simulink model "pFIR_Testing"  (R2019b)
settings: Solver=FixedStepDiscrete  StartTime=0.0  StopTime=stop_time  RelTol=1e-3
InitFcn:
  | pwd
  | sm_callback_init
StopFcn:
  | sm_callback_stop
values from neighbouring files (symbols this model uses):
  mp = sm_stop_process_output(mp)    [sm_callback_stop.m]
libraries: simulink x3, FPGA_Open_Speech_Tools x2
settings Model: Creator=Ross  LastModifiedBy=Balad
settings DataIOCC: ReturnWorkspaceOutputs=off
settings OptimizationCC: BlockReduction=off  ConditionallyExecuteInputs=off  DefaultParameterBehavior=Inlined
settings DebuggingCC: ReadBeforeWriteMsg=DisableAll  WriteAfterWriteMsg=DisableAll  WriteAfterReadMsg=DisableAll  AlgebraicLoopMsg=error  MultiTaskDSMMsg=none  SingleTaskRateTransMsg=error  PregeneratedLibrarySubsystemCodeDiagnostic=none  ArithmeticOperatorsInVariantConditions=warning
settings HardwareCC: ProdBitPerPointer=32  ProdBitPerSizeT=32  ProdBitPerPtrDiffT=32  ProdLargestAtomicFloat=None  ProdIntDivRoundTo=Undefined  ProdEndianess=Unspecified  ProdWordSize=32  ProdHWDeviceType=ASIC/FPGA->ASIC/FPGA  TargetBitPerPointer=64  TargetBitPerSizeT=64  TargetBitPerPtrDiffT=64  TargetLongLongMode=on  TargetIntDivRoundTo=Zero  TargetEndianess=LittleEndian  TargetWordSize=64  TargetHWDeviceType=Custom Processor->MATLAB Host Computer  ProdEqTarget=off
settings ModelReferenceCC: UpdateModelReferenceTargets=IfOutOfDate
settings SFSimCC: SFSimEcho=off  SimUseLocalCustomCode=off  CustomCodeUndefinedFunction=UseInterfaceOnly
settings RTWCC: RTWUseLocalCustomCode=off

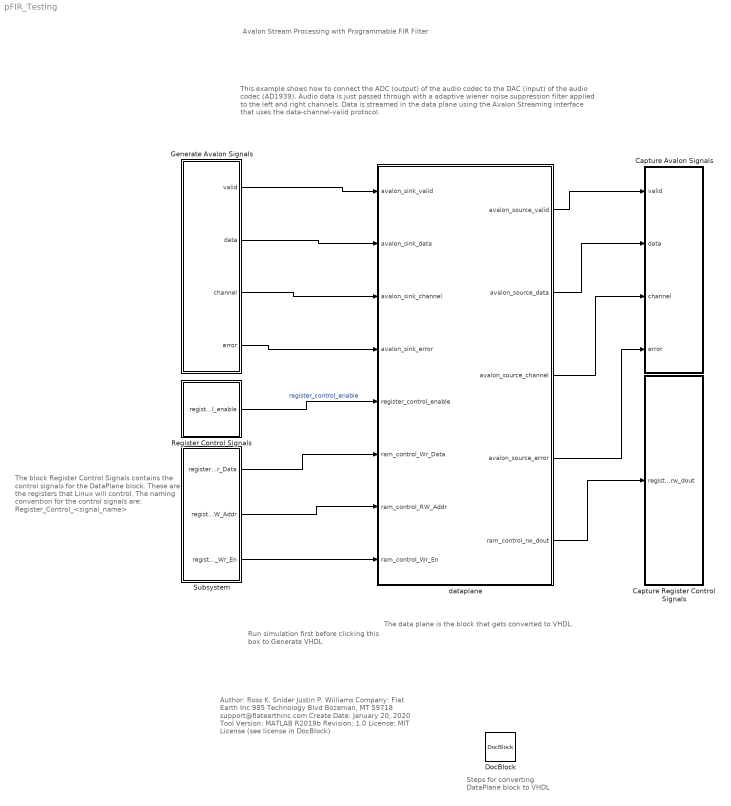
== system pFIR_Testing ==
  note: The data plane is the block that gets converted to VHDL.
  note: Author:          Ross K. Snider
      |                      Justin P. Williams
      | Company:     Flat Earth Inc
      |                       985 Technology Blvd
      |                       Bozeman, MT 59718
      |                       support@flatearthinc.com
      | Create Date:  January 20, 2020
      | Tool Version:  MATLAB R2019b
      | Revision:        1.0
      | License:          MIT License (see license in DocBlock)
  note: This example shows how to connect the ADC (output) of the audio codec to the DAC (input) of the audio codec (AD1939). Audio data is just passed through with a adaptive wiener noise suppression filter applied to the left and right channels. Data is streamed in the data plane using the Avalon Streaming interface that uses the data-channel-valid protocol.
  note: Steps for converting
      | DataPlane block
      | to VHDL
  note: Avalon Stream Processing
      | with Programmable FIR Filter
  note: Run simulation first
      | before clicking this box to
      | Generate VHDL
  note: The block Register Control Signals contains
      | the control signals for the DataPlane block.
      | These are the registers that Linux will control.
      | The naming convention for the control
      | signals are:  Register_Control_<signal_name>
  Capture Avalon Signals : Subsystem
  Capture Register Control Signals : Subsystem
  DocBlock : simulink/Model-Wide Utilities/DocBlock  DocumentType=HTML
  Generate Avalon Signals : Subsystem
  Register Control Signals : Subsystem
  Subsystem : Subsystem
  dataplane : Subsystem  TreatAsAtomicUnit=on
  wires:
  Generate Avalon Signals/2(data) -> dataplane/2(avalon_sink_data)
  Generate Avalon Signals/1(valid) -> dataplane/1(avalon_sink_valid)
  Generate Avalon Signals/3(channel) -> dataplane/3(avalon_sink_channel)
  Generate Avalon Signals/4(error) -> dataplane/4(avalon_sink_error)
  dataplane/2(avalon_source_data) -> Capture Avalon Signals/2(data)
  dataplane/1(avalon_source_valid) -> Capture Avalon Signals/1(valid)
  dataplane/3(avalon_source_channel) -> Capture Avalon Signals/3(channel)
  dataplane/4(avalon_source_error) -> Capture Avalon Signals/4(error)
  Register Control Signals/1(register_control_enable) -> dataplane/5(register_control_enable)  "register_control_enable"
  Subsystem/1(register_control_Wr_Data) -> dataplane/6(ram_control_Wr_Data)
  Subsystem/2(register_control_RW_Addr) -> dataplane/7(ram_control_RW_Addr)
  Subsystem/3(register_control_Wr_En) -> dataplane/8(ram_control_Wr_En)
  dataplane/5(ram_control_rw_dout) -> Capture Register Control Signals/1(register_control_rw_dout)

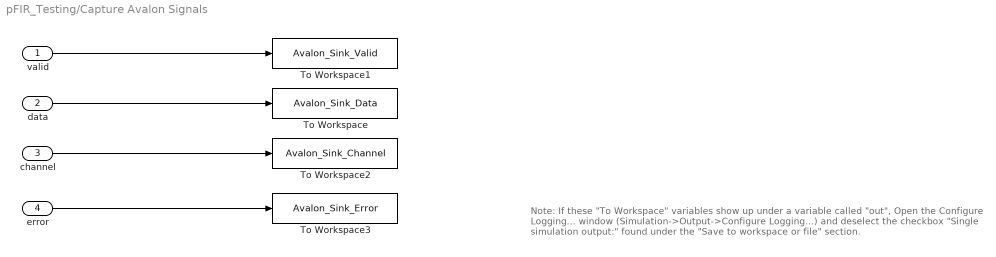
== system pFIR_Testing/Capture Avalon Signals ==
  note: Note:  If these "To Workspace" variables show up under a variable called "out",
      | Open the Configure Logging... window (Simulation->Output->Configure Logging...)
      | and deselect the checkbox "Single simulation output:" found under the "Save to workspace or file" section.
  valid : Inport
  data : Inport  Port=2
  channel : Inport  Port=3
  error : Inport  Port=4
  To Workspace : ToWorkspace  VariableName=Avalon_Sink_Data  SaveFormat=Timeseries  SampleTime=-1
  To Workspace1 : ToWorkspace  VariableName=Avalon_Sink_Valid  SaveFormat=Timeseries  SampleTime=-1
  To Workspace2 : ToWorkspace  VariableName=Avalon_Sink_Channel  SaveFormat=Timeseries  SampleTime=-1
  To Workspace3 : ToWorkspace  VariableName=Avalon_Sink_Error  SaveFormat=Timeseries  SampleTime=-1
  wires:
  data/1 -> To Workspace/1
  valid/1 -> To Workspace1/1
  error/1 -> To Workspace3/1
  channel/1 -> To Workspace2/1

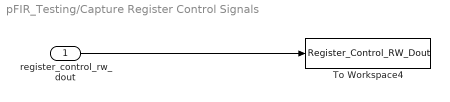
== system pFIR_Testing/Capture Register Control Signals ==
  register_control_rw_dout : Inport
  To Workspace4 : ToWorkspace  VariableName=Register_Control_RW_Dout  SaveFormat=Timeseries  SampleTime=-1
  wires:
  register_control_rw_dout/1 -> To Workspace4/1

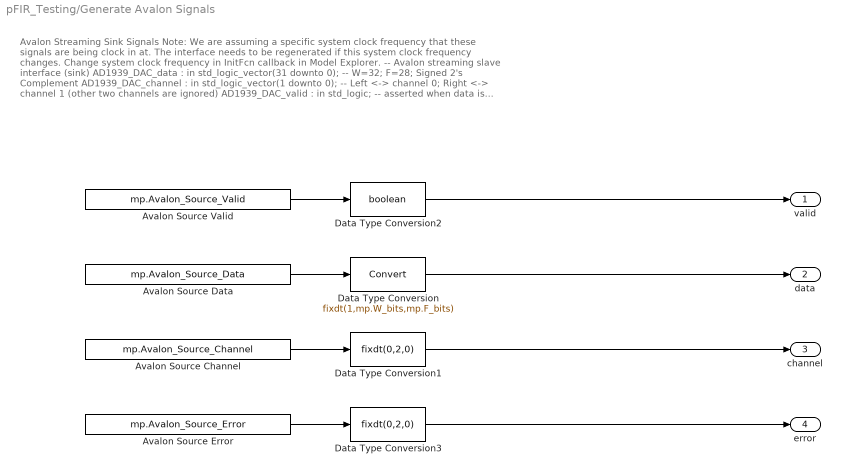
== system pFIR_Testing/Generate Avalon Signals ==
  note: Avalon Streaming Sink Signals
      | Note: We are assuming a specific system clock frequency that these signals are being clock in at.
      | The interface needs to be regenerated if this system clock frequency changes. Change system clock frequency in InitFcn callback in Model Explorer.
      |
      | -- Avalon streaming slave interface (sink)
      | AD1939_DAC_data : in std_logic_vector(31 downto 0); -- W=32; F=28; Signed 2's Complement
      | AD1939_DAC_channel : in std_logic_vector(1 downto 0); -- Left <-> channel 0; Right <-> channel 1 (other two channels are ignored)
      | AD1939_DAC_valid : in std_logic; -- asserted when data is valid
      | AD1939_DAC_error : in std_logic_vector(1 downto 0) -- error channel is ignored, assumed to be error free at this point
      |
      | For more information on the data-channel-valid protocol, s ee chapter 5 in Intel's Avalon Interfaced Specification (p. 40) at https://www.intel.com/content/dam/www/programmable/us/en/pdfs/literature/manual/mnl_avalon_spec.pdf
  Avalon Source Channel : FromWorkspace  VariableName=mp.Avalon_Source_Channel  OutDataTypeStr=double  SampleTime=mp.Ts_system
  "Avalon Source Data " : FromWorkspace  VariableName=mp.Avalon_Source_Data  OutDataTypeStr=double  SampleTime=mp.Ts_system
  Avalon Source Error : FromWorkspace  VariableName=mp.Avalon_Source_Error  OutDataTypeStr=double  SampleTime=mp.Ts_system
  Avalon Source Valid : FromWorkspace  VariableName=mp.Avalon_Source_Valid  OutDataTypeStr=double  SampleTime=mp.Ts_system
  Data Type Conversion : DataTypeConversion  OutDataTypeStr=fixdt(1,mp.W_bits,mp.F_bits)
  Data Type Conversion1 : DataTypeConversion  OutDataTypeStr=fixdt(0,2,0)
  Data Type Conversion2 : DataTypeConversion  OutDataTypeStr=boolean
  Data Type Conversion3 : DataTypeConversion  OutDataTypeStr=fixdt(0,2,0)
  valid : Outport  VectorParamsAs1DForOutWhenUnconnected=off
  data : Outport  Port=2  VectorParamsAs1DForOutWhenUnconnected=off
  channel : Outport  Port=3  VectorParamsAs1DForOutWhenUnconnected=off
  error : Outport  Port=4  VectorParamsAs1DForOutWhenUnconnected=off
  wires:
  Data Type Conversion1/1 -> channel/1
  Data Type Conversion2/1 -> valid/1
  Avalon Source Error/1 -> Data Type Conversion3/1
  Data Type Conversion/1 -> data/1
  Avalon Source Valid/1 -> Data Type Conversion2/1
  Data Type Conversion3/1 -> error/1
  Avalon Source Channel/1 -> Data Type Conversion1/1
  "Avalon Source Data "/1 -> Data Type Conversion/1

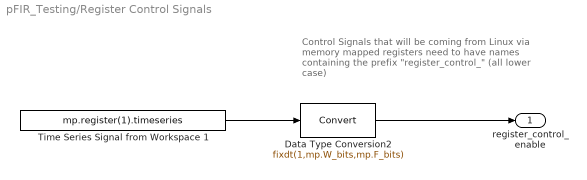
== system pFIR_Testing/Register Control Signals ==
  note: Control Signals that will be coming from Linux via
      | memory mapped registers need to have names
      | containing the prefix "register_control_"
      | (all lower case)
  Data Type Conversion2 : DataTypeConversion  OutDataTypeStr=fixdt(1,mp.W_bits,mp.F_bits)
  Time Series Signal from Workspace 1 : FromWorkspace  VariableName=mp.register(1).timeseries  OutDataTypeStr=double  SampleTime=mp.Ts_system  OutputAfterFinalValue=Holding final value
  register_control_enable : Outport  VectorParamsAs1DForOutWhenUnconnected=off
  wires:
  Time Series Signal from Workspace 1/1 -> Data Type Conversion2/1
  Data Type Conversion2/1 -> register_control_enable/1

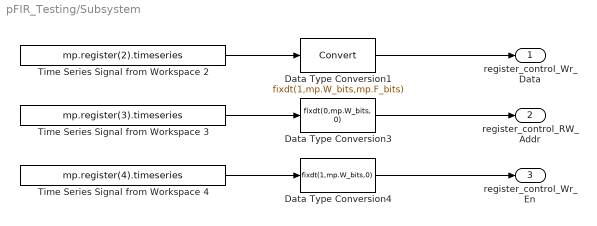
== system pFIR_Testing/Subsystem ==
  Data Type Conversion1 : DataTypeConversion  OutDataTypeStr=fixdt(1,mp.W_bits,mp.F_bits)
  Data Type Conversion3 : DataTypeConversion  OutDataTypeStr=fixdt(0,mp.W_bits, 0)
  Data Type Conversion4 : DataTypeConversion  OutDataTypeStr=fixdt(1,mp.W_bits,0)
  Time Series Signal from Workspace 2 : FromWorkspace  VariableName=mp.register(2).timeseries  OutDataTypeStr=double  SampleTime=mp.Ts_system
  Time Series Signal from Workspace 3 : FromWorkspace  VariableName=mp.register(3).timeseries  OutDataTypeStr=double  SampleTime=mp.Ts_system
  Time Series Signal from Workspace 4 : FromWorkspace  VariableName=mp.register(4).timeseries  OutDataTypeStr=double  SampleTime=mp.Ts_system
  register_control_Wr_Data : Outport  VectorParamsAs1DForOutWhenUnconnected=off
  register_control_RW_Addr : Outport  Port=2  VectorParamsAs1DForOutWhenUnconnected=off
  register_control_Wr_En : Outport  Port=3  VectorParamsAs1DForOutWhenUnconnected=off
  wires:
  Data Type Conversion1/1 -> register_control_Wr_Data/1
  Time Series Signal from Workspace 4/1 -> Data Type Conversion4/1
  Data Type Conversion3/1 -> register_control_RW_Addr/1
  Data Type Conversion4/1 -> register_control_Wr_En/1
  Time Series Signal from Workspace 3/1 -> Data Type Conversion3/1
  Time Series Signal from Workspace 2/1 -> Data Type Conversion1/1

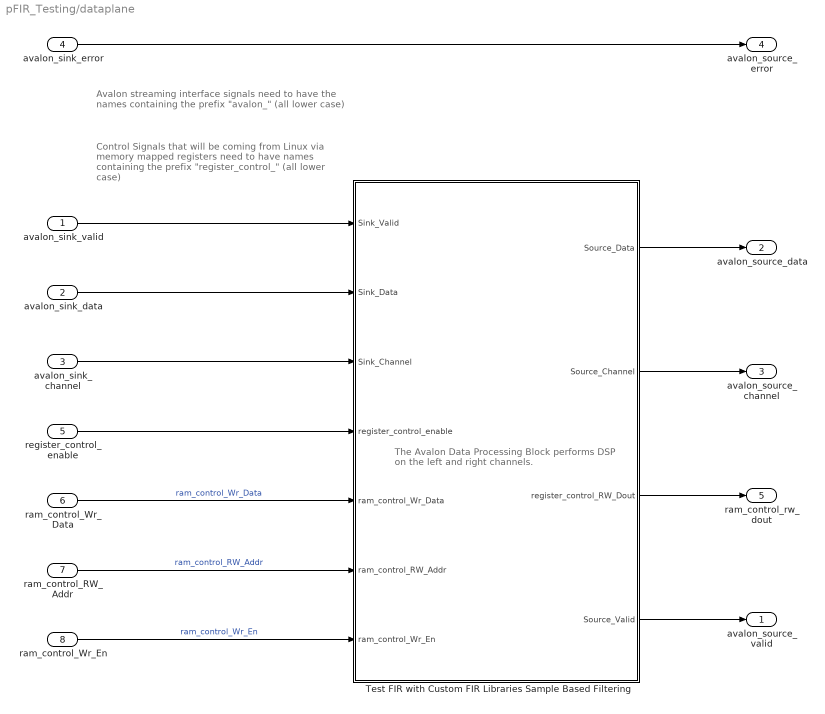
== system pFIR_Testing/dataplane ==
  note: Control Signals that will be coming from Linux via
      | memory mapped registers need to have names
      | containing the prefix "register_control_"
      | (all lower case)
  note: The Avalon Data Processing Block
      | performs DSP on the left and right channels.
  note: Avalon streaming interface signals need to have the
      | names containing the prefix "avalon_"
      | (all lower case)
  avalon_sink_valid : Inport
  avalon_sink_data : Inport  Port=2
  avalon_sink_channel : Inport  Port=3
  avalon_sink_error : Inport  Port=4
  register_control_enable : Inport  Port=5
  ram_control_Wr_Data : Inport  Port=6
  ram_control_RW_Addr : Inport  Port=7
  ram_control_Wr_En : Inport  Port=8
  Test FIR with Custom FIR Libraries Sample Based Filtering : Subsystem
  avalon_source_valid : Outport  VectorParamsAs1DForOutWhenUnconnected=off
  avalon_source_data : Outport  Port=2  VectorParamsAs1DForOutWhenUnconnected=off
  avalon_source_channel : Outport  Port=3  VectorParamsAs1DForOutWhenUnconnected=off
  avalon_source_error : Outport  Port=4  VectorParamsAs1DForOutWhenUnconnected=off
  ram_control_rw_dout : Outport  Port=5  VectorParamsAs1DForOutWhenUnconnected=off
  wires:
  avalon_sink_error/1 -> avalon_source_error/1
  Test FIR with Custom FIR Libraries Sample Based Filtering/1(Source_Data) -> avalon_source_data/1
  avalon_sink_valid/1 -> Test FIR with Custom FIR Libraries Sample Based Filtering/1(Sink_Valid)
  avalon_sink_data/1 -> Test FIR with Custom FIR Libraries Sample Based Filtering/2(Sink_Data)
  Test FIR with Custom FIR Libraries Sample Based Filtering/2(Source_Channel) -> avalon_source_channel/1
  avalon_sink_channel/1 -> Test FIR with Custom FIR Libraries Sample Based Filtering/3(Sink_Channel)
  register_control_enable/1 -> Test FIR with Custom FIR Libraries Sample Based Filtering/4(register_control_enable)
  ram_control_Wr_Data/1 -> Test FIR with Custom FIR Libraries Sample Based Filtering/5(ram_control_Wr_Data)  "ram_control_Wr_Data"
  ram_control_RW_Addr/1 -> Test FIR with Custom FIR Libraries Sample Based Filtering/6(ram_control_RW_Addr)  "ram_control_RW_Addr"
  ram_control_Wr_En/1 -> Test FIR with Custom FIR Libraries Sample Based Filtering/7(ram_control_Wr_En)  "ram_control_Wr_En"
  Test FIR with Custom FIR Libraries Sample Based Filtering/3(register_control_RW_Dout) -> ram_control_rw_dout/1
  Test FIR with Custom FIR Libraries Sample Based Filtering/4(Source_Valid) -> avalon_source_valid/1

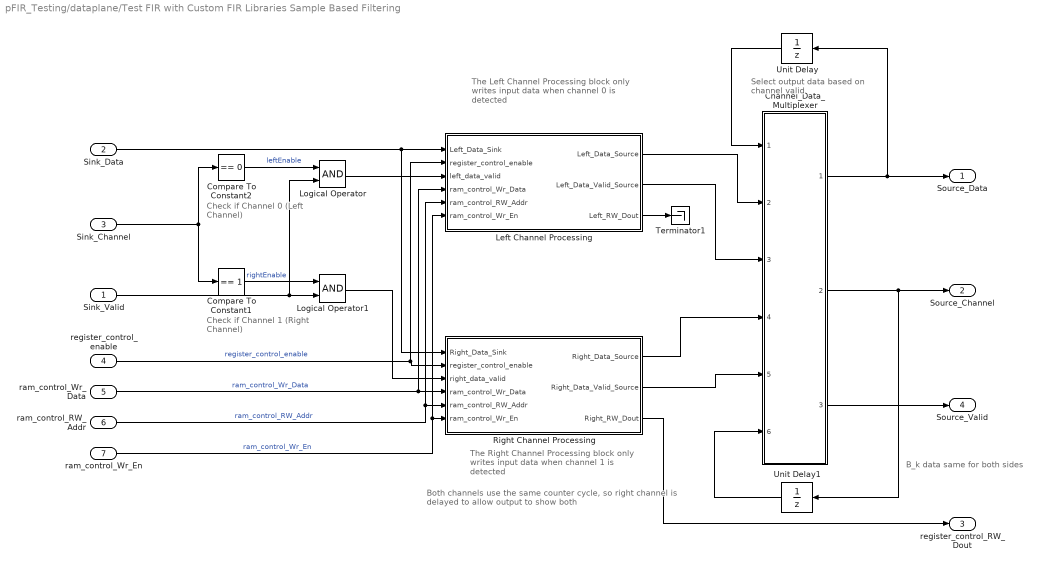
== system pFIR_Testing/dataplane/Test FIR with Custom FIR Libraries Sample Based Filtering ==
  note: B_k data same for both sides
  note: Both channels use the same counter cycle, so right channel
      | is delayed to allow output to show both
  note: The Left Channel Processing block
      | only writes input data when channel 0
      | is detected
  note: The Right Channel Processing block
      | only writes input data when channel 1
      | is detected
  note: Check if Channel 0
      | (Left Channel)
  note: Select output data
      | based on channel valid
  note: Check if Channel 1
      | (Right Channel)
  Sink_Valid : Inport
  Sink_Data : Inport  Port=2
  Sink_Channel : Inport  Port=3
  register_control_enable : Inport  Port=4
  ram_control_Wr_Data : Inport  Port=5
  ram_control_RW_Addr : Inport  Port=6
  ram_control_Wr_En : Inport  Port=7
  Channel_Data_Multiplexer : MATLAB Function  TreatAsAtomicUnit=on
  Compare To Constant1 : simulink/Logic and Bit Operations/Compare To Constant  relop===  const=1  OutDataTypeStr=boolean
  Compare To Constant2 : simulink/Logic and Bit Operations/Compare To Constant  relop===  const=0  OutDataTypeStr=boolean
  Left Channel Processing : Subsystem  TreatAsAtomicUnit=on
  Logical Operator : Logic  AllPortsSameDT=off  OutDataTypeStr=boolean
  Logical Operator1 : Logic  AllPortsSameDT=off  OutDataTypeStr=boolean
  Right Channel Processing : Subsystem  TreatAsAtomicUnit=on
  Terminator1 : Terminator
  Unit Delay : UnitDelay  SampleTime=-1  HasFrameUpgradeWarning=on
  Unit Delay1 : UnitDelay  SampleTime=-1  HasFrameUpgradeWarning=on
  Source_Data : Outport  InitialOutput=0  VectorParamsAs1DForOutWhenUnconnected=off
  Source_Channel : Outport  Port=2  InitialOutput=0  VectorParamsAs1DForOutWhenUnconnected=off
  register_control_RW_Dout : Outport  Port=3  InitialOutput=0  VectorParamsAs1DForOutWhenUnconnected=off
  Source_Valid : Outport  Port=4  InitialOutput=0  VectorParamsAs1DForOutWhenUnconnected=off
  wires:
  Left Channel Processing/1("Left_Data_Source ") -> Channel_Data_Multiplexer/2(leftData)
  Channel_Data_Multiplexer/1(sourceData) -> Unit Delay/1, Source_Data/1
  Compare To Constant2/1 -> Logical Operator/1  "leftEnable"
  Sink_Data/1 -> Left Channel Processing/1(Left_Data_Sink), Right Channel Processing/1(Right_Data_Sink)
  Sink_Channel/1 -> Compare To Constant1/1, Compare To Constant2/1
  Compare To Constant1/1 -> Logical Operator1/1  "rightEnable"
  register_control_enable/1 -> Right Channel Processing/2(register_control_enable), Left Channel Processing/2(register_control_enable)  "register_control_enable"
  Left Channel Processing/2(Left_Data_Valid_Source) -> Channel_Data_Multiplexer/3(leftValid)
  Sink_Valid/1 -> Logical Operator/2, Logical Operator1/2
  Logical Operator/1 -> Left Channel Processing/3(left_data_valid)
  Logical Operator1/1 -> Right Channel Processing/3(right_data_valid)
  ram_control_Wr_Data/1 -> Left Channel Processing/4(ram_control_Wr_Data), Right Channel Processing/4(ram_control_Wr_Data)  "ram_control_Wr_Data"
  ram_control_RW_Addr/1 -> Left Channel Processing/5(ram_control_RW_Addr), Right Channel Processing/5(ram_control_RW_Addr)  "ram_control_RW_Addr"
  ram_control_Wr_En/1 -> Left Channel Processing/6(ram_control_Wr_En), Right Channel Processing/6(ram_control_Wr_En)  "ram_control_Wr_En"
  Left Channel Processing/3(Left_RW_Dout) -> Terminator1/1
  Right Channel Processing/3(Right_RW_Dout) -> register_control_RW_Dout/1
  Right Channel Processing/1("Right_Data_Source ") -> Channel_Data_Multiplexer/4(rightData)
  Right Channel Processing/2(Right_Data_Valid_Source) -> Channel_Data_Multiplexer/5(rightValid)
  Channel_Data_Multiplexer/2(sourceChannel) -> Source_Channel/1, Unit Delay1/1
  Channel_Data_Multiplexer/3(sourceValid) -> Source_Valid/1
  Unit Delay/1 -> Channel_Data_Multiplexer/1(dataPrev)
  Unit Delay1/1 -> Channel_Data_Multiplexer/6(chanPrev)

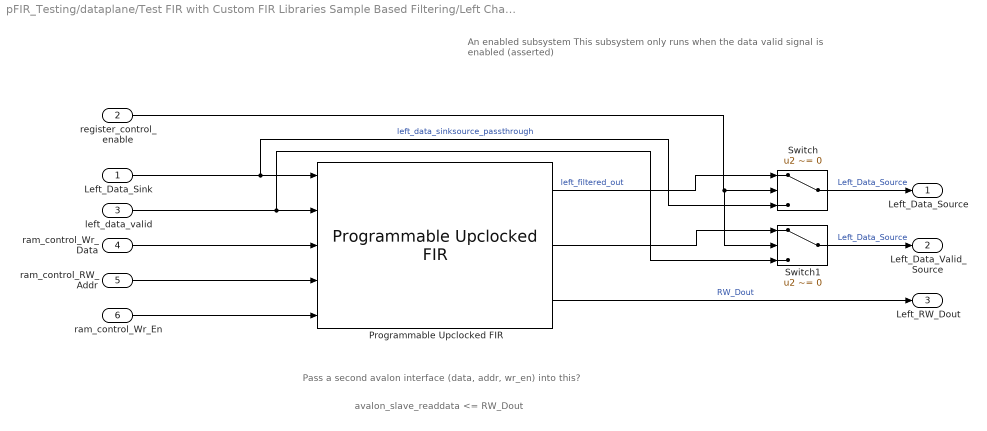
== system pFIR_Testing/dataplane/Test FIR with Custom FIR Libraries Sample Based Filtering/Left Channel Processing ==
  note: avalon_slave_readdata <= RW_Dout
  note: Pass a second avalon interface (data, addr, wr_en) into this?
  note: An enabled subsystem
      | This subsystem only runs when the data valid signal is enabled (asserted)
  Left_Data_Sink : Inport
  register_control_enable : Inport  Port=2
  left_data_valid : Inport  Port=3
  ram_control_Wr_Data : Inport  Port=4
  ram_control_RW_Addr : Inport  Port=5
  ram_control_Wr_En : Inport  Port=6
  Programmable Upclocked FIR : FPGA_Open_Speech_Tools/Programmable Upclocked FIR  b_k=mp.LPF_1000  Ts=mp.Ts  Ts_system=mp.Ts_system  rotationDelay=0  W_bits=32  F_bits=28
  Switch : Switch  Criteria=u2 ~= 0  Threshold=1
  Switch1 : Switch  Criteria=u2 ~= 0  Threshold=1
  "Left_Data_Source " : Outport  InitialOutput=0  VectorParamsAs1DForOutWhenUnconnected=off
  Left_Data_Valid_Source : Outport  Port=2  InitialOutput=0  VectorParamsAs1DForOutWhenUnconnected=off
  Left_RW_Dout : Outport  Port=3  InitialOutput=0  VectorParamsAs1DForOutWhenUnconnected=off
  wires:
  register_control_enable/1 -> Switch1/2, Switch/2
  Programmable Upclocked FIR/1 -> Switch/1  "left_filtered_out"
  Left_Data_Sink/1 -> Programmable Upclocked FIR/1, Switch/3  "left_data_sinksource_passthrough"
  Switch/1 -> "Left_Data_Source "/1  "Left_Data_Source"
  left_data_valid/1 -> Switch1/3, Programmable Upclocked FIR/2
  Programmable Upclocked FIR/2 -> Switch1/1
  ram_control_Wr_Data/1 -> Programmable Upclocked FIR/3
  ram_control_RW_Addr/1 -> Programmable Upclocked FIR/4
  ram_control_Wr_En/1 -> Programmable Upclocked FIR/5
  Programmable Upclocked FIR/3 -> Left_RW_Dout/1  "RW_Dout"
  Switch1/1 -> Left_Data_Valid_Source/1  "Left_Data_Source"

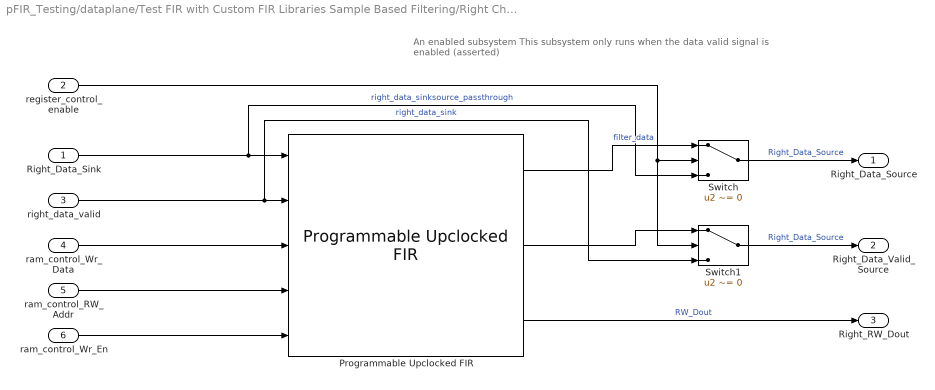
== system pFIR_Testing/dataplane/Test FIR with Custom FIR Libraries Sample Based Filtering/Right Channel Processing ==
  note: An enabled subsystem
      | This subsystem only runs when the data valid signal is enabled (asserted)
  Right_Data_Sink : Inport
  register_control_enable : Inport  Port=2
  right_data_valid : Inport  Port=3
  ram_control_Wr_Data : Inport  Port=4
  ram_control_RW_Addr : Inport  Port=5
  ram_control_Wr_En : Inport  Port=6
  Programmable Upclocked FIR : FPGA_Open_Speech_Tools/Programmable Upclocked FIR  b_k=mp.LPF_1000  Ts=mp.Ts  Ts_system=mp.Ts_system  rotationDelay=0  W_bits=32  F_bits=28
  Switch : Switch  Criteria=u2 ~= 0  Threshold=1
  Switch1 : Switch  Criteria=u2 ~= 0  Threshold=1
  "Right_Data_Source " : Outport  OutDataTypeStr=fixdt(1, mp.W_bits, mp.F_bits)  InitialOutput=0  VectorParamsAs1DForOutWhenUnconnected=off  LockScale=on
  Right_Data_Valid_Source : Outport  Port=2  InitialOutput=0  VectorParamsAs1DForOutWhenUnconnected=off
  Right_RW_Dout : Outport  Port=3  InitialOutput=0  VectorParamsAs1DForOutWhenUnconnected=off
  wires:
  right_data_valid/1 -> Switch1/3, Programmable Upclocked FIR/2  "right_data_sink"
  Switch/1 -> "Right_Data_Source "/1  "Right_Data_Source"
  Right_Data_Sink/1 -> Switch/3, Programmable Upclocked FIR/1  "right_data_sinksource_passthrough"
  Programmable Upclocked FIR/1 -> Switch/1  "filter_data"
  register_control_enable/1 -> Switch1/2, Switch/2
  ram_control_Wr_Data/1 -> Programmable Upclocked FIR/3
  ram_control_RW_Addr/1 -> Programmable Upclocked FIR/4
  ram_control_Wr_En/1 -> Programmable Upclocked FIR/5
  Programmable Upclocked FIR/3 -> Right_RW_Dout/1  "RW_Dout"
  Programmable Upclocked FIR/2 -> Switch1/1
  Switch1/1 -> Right_Data_Valid_Source/1  "Right_Data_Source"

== matlab function pFIR_Testing/dataplane/Test FIR with Custom FIR Libraries Sample Based Filtering/Channel_Data_Multiplexer ==
  data: dataPrev input fixdt(1,mp.W_bits,mp.F_bits); sourceData output fixdt(1,mp.W_bits,mp.F_bits); leftData input fixdt(1,mp.W_bits,mp.F_bits); sourceChannel output; leftValid input boolean; rightData input fixdt(1,mp.W_bits,mp.F_bits); rightValid input boolean; sourceValid output; chanPrev input fixdt(0,2,0)
function [sourceData, sourceChannel, sourceValid] = fcn(dataPrev, leftData, leftValid, rightData, rightValid, chanPrev)
%#codegen
    if(leftValid)               % left channel ready
        sourceData = leftData;
        sourceChannel = fi(0, 0, 2, 0); 
        sourceValid = fi(1, 0, 1, 0);
    elseif(rightValid)          % right channel ready 
        sourceData = rightData;
        sourceChannel = fi(1, 0, 2, 0);
        sourceValid = fi(1, 0, 1, 0);
    else                        % neither channel output is ready
        sourceData = dataPrev;
        sourceChannel = chanPrev;
        sourceValid = fi(0, 0, 1, 0);
    end
end
